simulink model "InteriorLight"  (R2021b)
settings: Solver=VariableStepAuto  StartTime=0.0  StopTime=10.0  RelTol=1e-3
settings Model: Creator=AGM4GA  LastModifiedBy=AGM4GA

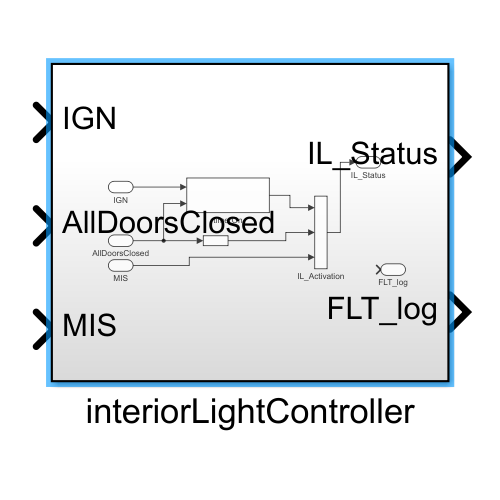
[thumbnail: Simulink's stored preview of the top-level diagram]
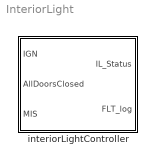
== system InteriorLight ==
  interiorLightController : Subsystem

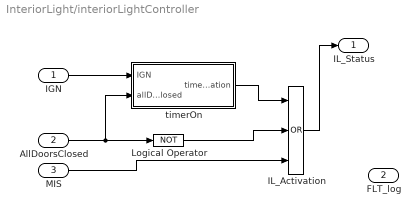
== system InteriorLight/interiorLightController ==
  IGN : Inport
  AllDoorsClosed : Inport  Port=2
  MIS : Inport  Port=3
  IL_Activation : Logic  Operator=OR  Inputs=3  AllPortsSameDT=off  OutDataTypeStr=boolean
  Logical Operator : Logic  Operator=NOT  AllPortsSameDT=off  OutDataTypeStr=boolean
  timerOn : Subsystem
  IL_Status : Outport
  FLT_log : Outport  Port=2
  wires:
  MIS/1 -> IL_Activation/3
  IL_Activation/1 -> IL_Status/1
  Logical Operator/1 -> IL_Activation/2
  timerOn/1(timerActivation) -> IL_Activation/1
  AllDoorsClosed/1 -> timerOn/2(allDoorsClosed), Logical Operator/1
  IGN/1 -> timerOn/1(IGN)

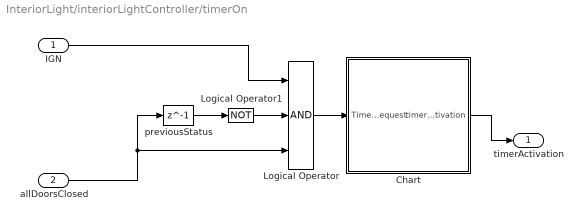
== system InteriorLight/interiorLightController/timerOn ==
  IGN : Inport
  allDoorsClosed : Inport  Port=2
  Chart : Stateflow chart  TreatAsAtomicUnit=on
  Logical Operator : Logic  Inputs=3  AllPortsSameDT=off  OutDataTypeStr=boolean
  Logical Operator1 : Logic  Operator=NOT  AllPortsSameDT=off  OutDataTypeStr=boolean
  previousStatus : Delay  DelayLength=1  InputProcessing=Columns as channels (frame based)
  timerActivation : Outport
  wires:
  IGN/1 -> Logical Operator/1
  allDoorsClosed/1 -> Logical Operator/3, previousStatus/1
  previousStatus/1 -> Logical Operator1/1
  Logical Operator1/1 -> Logical Operator/2
  Logical Operator/1 -> Chart/1(TimerRequest)
  Chart/1(timerActivation) -> timerActivation/1

== stateflow chart InteriorLight/interiorLightController/timerOn/Chart ==
  (junction 15) -> (junction 8) [order 2]
  5 -> (junction 15)
  (junction 15) -> (junction 4) [order 1]
  (junction 4) -> (junction 8) [order 1] : [timer < TIME_LIMIT]
  (junction 4) -> (junction 7) [order 2] : {timerActivation =0;}
  (junction 8) -> (junction 12) : {timer = timer + 1;
      | timerActivation = 1;}
  (junction 12) -> (junction 7)
  data: TimerRequest input; timerActivation output
